simulink library "ayazGroundStation_cl"  (R2018b)
settings: Solver=VariableStepAuto  StartTime=0.0  StopTime=10.0  RelTol=1e-3
settings Model: Creator=mcobb  LastModifiedBy=mcobb

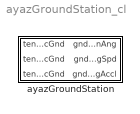
== system ayazGroundStation_cl ==
  ayazGroundStation : Subsystem

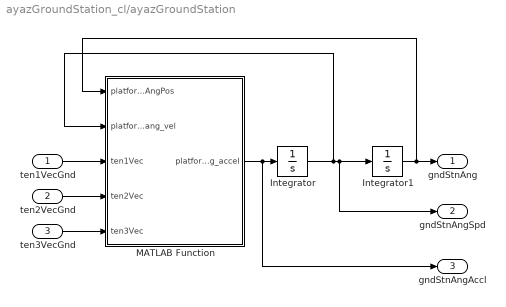
== system ayazGroundStation_cl/ayazGroundStation ==
  ten1VecGnd : Inport
  ten2VecGnd : Inport  Port=2
  ten3VecGnd : Inport  Port=3
  Integrator : Integrator
  Integrator1 : Integrator
  MATLAB Function : MATLAB Function  TreatAsAtomicUnit=on
  gndStnAng : Outport
  gndStnAngSpd : Outport  Port=2
  gndStnAngAccl : Outport  Port=3
  wires:
  ten1VecGnd/1 -> MATLAB Function/3(ten1Vec)
  ten2VecGnd/1 -> MATLAB Function/4(ten2Vec)
  ten3VecGnd/1 -> MATLAB Function/5(ten3Vec)
  Integrator1/1 -> MATLAB Function/1(platformAngPos), gndStnAng/1
  Integrator/1 -> Integrator1/1, gndStnAngSpd/1, MATLAB Function/2(platform_ang_vel)
  MATLAB Function/1(platform_ang_accel) -> gndStnAngAccl/1, Integrator/1

== matlab function ayazGroundStation_cl/ayazGroundStation/MATLAB Function ==
  data: platformAngPos input; platform_ang_vel input; ten1Vec input; ten2Vec input; ten3Vec input; platform_ang_accel output; sim_param parameter
function platform_ang_accel = fcn(platformAngPos,platform_ang_vel,ten1Vec,ten2Vec,ten3Vec,sim_param)


pCo = [cos(platformAngPos) sin(platformAngPos) 0; -sin(platformAngPos) cos(platformAngPos) 0; 0 0 1];

P_Izz = sim_param.platform_param.platform_Izz;
cp = sim_param.platform_param.platform_damping;

T_o_ext =   cross(sim_param.tether_imp_nodes.R1n_cm,(pCo*ten1Vec)) + ...
            cross(sim_param.tether_imp_nodes.R2n_cm,(pCo*ten2Vec)) + ...
            cross(sim_param.tether_imp_nodes.R3n_cm,(pCo*ten3Vec));

platform_ang_accel = (T_o_ext(end)/P_Izz) - cp*platform_ang_vel;

end
